simulink model "Lab4_4"  (R2015a)
settings: Solver=ode3  StartTime=0.0  StopTime=inf  RelTol=1e-3
settings Model: SimulationMode=external  ExtModeTrigDuration=2  Creator=007313527  LastModifiedBy=007313527
settings OptimizationCC: OptimizeModelRefInitCode=on  LifeSpan=1
settings DebuggingCC: UnderspecifiedInitializationDetection=Classic  MergeDetectMultiDrivingBlocksExec=none
settings HardwareCC: ProdBitPerInt=16  ProdBitPerPointer=8  ProdIntDivRoundTo=Zero  ProdEndianess=LittleEndian  ProdWordSize=8  ProdHWDeviceType=Atmel->AVR
settings RTWCC: SystemTargetFile=realtime.tlc  GenerateMakefile=off  TemplateMakefile=realtime.tmf  Description=Run on Target Hardware  RTWVerbose=off
settings ERTTargetCC: CombineOutputUpdateFcns=off  ExtModeTransport=3  ExtModeMexFile=ext_serial_win32_comm_rtt  ExtModeMexArgs=0 1 9600  ERTSrcFileBannerTemplate=realtime_code_template.cgt  ERTHdrFileBannerTemplate=realtime_code_template.cgt  ERTDataSrcFileTemplate=realtime_code_template.cgt  ERTDataHdrFileTemplate=realtime_code_template.cgt  ERTCustomFileTemplate=realtime_file_process.tlc

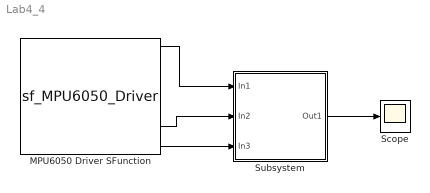
== system Lab4_4 ==
  MPU6050 Driver SFunction : S-Function  InitFcn=try, set_param(gcb,'FunctionName','sf_MPU6050_Driver'), end  FunctionName=sf_MPU6050_Driver  SFunctionModules=sf_MPU6050_Driver_wrapper  mask(S-Function Builder){}
      mask help: Simulink:masks:SFunctionBuilder_MD
      mask init:
      | val = [[.9  0.75 0.75 1 1 .9 .9 1]',[1 1 0.75 0.75 .9 .9 1 .9]'];try , sys = get_param(gcb,'SfunBuilderFcnName');if isempty(sys), sys = get_param(gcb,'FunctionName'); end,catch, sys = get_param(gcb,'FunctionName'); end
      settings: CopyFcn=set_param(gcbh,'LinkStatus','none')  PreSaveFcn=try, set_param(gcb,'FunctionName','sf_MPU6050_Driver'), end  OpenFcn=sfunctionwizard(gcbh)
      mask Display: plot(val(:,1),val(:,2)),disp(sys), port_label('output',1,'x_vel'), port_label('output',2,'y_vel'), port_label('output',3,'z_vel'), port_label('output',4,'x_acc'), port_label('output',5,'y_acc'), port_label('output',6,'z_acc')
  Scope : Scope
      settings: TimeRange=10  YMin=-0.5  YMax=5.5
  Subsystem : Subsystem
  wires:
  MPU6050 Driver SFunction/1 -> Subsystem/1(In1)
  MPU6050 Driver SFunction/5 -> Subsystem/2(In2)
  MPU6050 Driver SFunction/6 -> Subsystem/3(In3)
  Subsystem/1(Out1) -> Scope/1

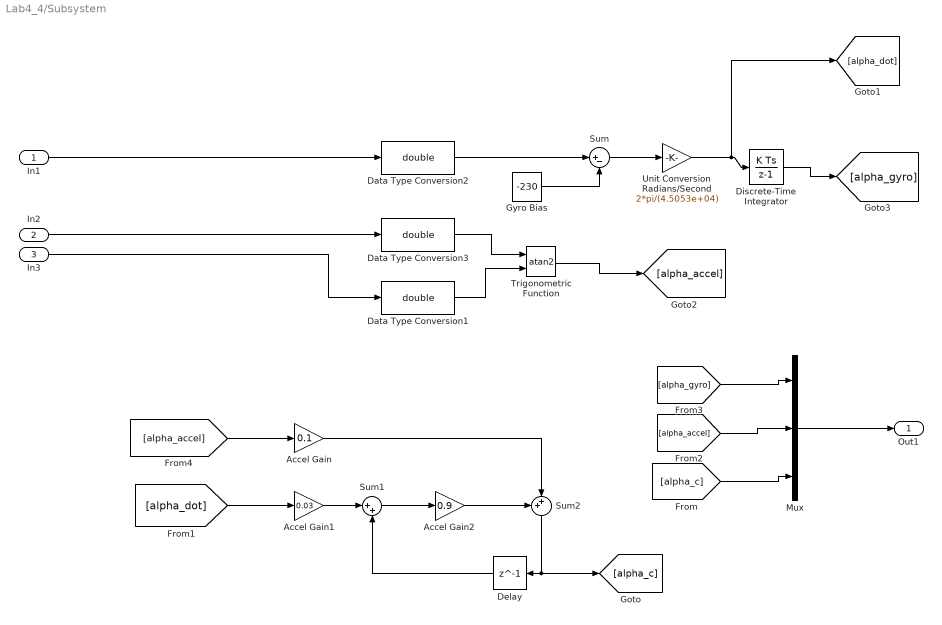
== system Lab4_4/Subsystem ==
  In1 : Inport
  In2 : Inport  Port=2
  In3 : Inport  Port=3
  Accel Gain : Gain  Gain=0.1
  Accel Gain1 : Gain  Gain=0.03
  Accel Gain2 : Gain  Gain=0.9
  Data Type Conversion1 : DataTypeConversion  OutDataTypeStr=double
  Data Type Conversion2 : DataTypeConversion  OutDataTypeStr=double
  Data Type Conversion3 : DataTypeConversion  OutDataTypeStr=double
  Delay : Delay  DelayLength=1  InitialCondition=0
  Discrete-Time Integrator : DiscreteIntegrator  InitialConditionSetting=State (most efficient)  SampleTime=-1
  Gyro Bias : Constant  Value=-230
  Mux : Mux  Inputs=3
  Sum : Sum  Inputs=|+-
  Sum1 : Sum  Inputs=|++
  Sum2 : Sum  Inputs=++|
  Trigonometric Function : Trigonometry  Operator=atan2
  Unit Conversion Radians/Second : Gain  Gain=2*pi/(4.5053e+04)
  Out1 : Outport
  wires:
  Data Type Conversion2/1 -> Sum/1
  Gyro Bias/1 -> Sum/2
  Unit Conversion Radians/Second/1 -> [alpha_dot], Discrete-Time Integrator/1
  [alpha_accel] -> Accel Gain/1
  In1/1 -> Data Type Conversion2/1
  Data Type Conversion3/1 -> Trigonometric Function/1
  In2/1 -> Data Type Conversion3/1
  Discrete-Time Integrator/1 -> [alpha_gyro]
  In3/1 -> Data Type Conversion1/1
  Trigonometric Function/1 -> [alpha_accel]
  Data Type Conversion1/1 -> Trigonometric Function/2
  Sum/1 -> Unit Conversion Radians/Second/1
  [alpha_dot] -> Accel Gain1/1
  Accel Gain1/1 -> Sum1/1
  Accel Gain2/1 -> Sum2/1
  Delay/1 -> Sum1/2
  Sum1/1 -> Accel Gain2/1
  Accel Gain/1 -> Sum2/2
  [alpha_gyro] -> Mux/1
  Mux/1 -> Out1/1
  [alpha_accel] -> Mux/2
  [alpha_c] -> Mux/3
  Sum2/1 -> [alpha_c], Delay/1
